simulink model "Subsystem"  (R2020a)
settings: Solver=FixedStepAuto  StartTime=0.0  StopTime=10.0  FixedStep=0.2  RelTol=1e-3
settings Model: Creator=Jake  LastModifiedBy=Jake
settings DataIOCC: SaveOutput=off  SaveTime=off

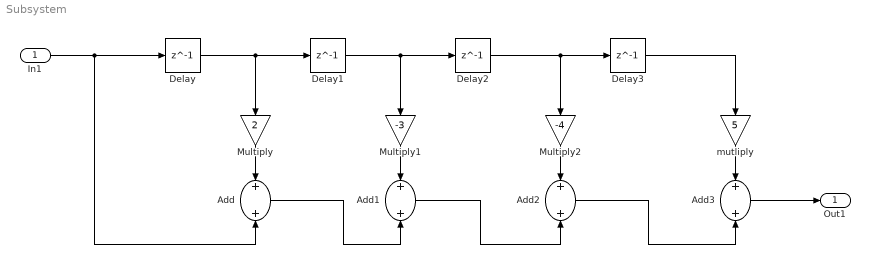
== system Subsystem ==
  In1 : Inport  OutDataTypeStr=double  PortDimensions=1  SampleTime=[0.20000000000000001,0]
  Add{,1..3} (4 alike) : Sum
  Delay{,1..3} (4 alike) : Delay  DelayLength=1
  Multiply : Gain  Gain=2
  Multiply1 : Gain  Gain=-3
  Multiply2 : Gain  Gain=-4
  mutliply : Gain  Gain=5
  Out1 : Outport  OutDataTypeStr=double  PortDimensions=1  SampleTime=[0.20000000000000001,0]
  wires:
  Multiply2/1 -> Add2/1
  Delay2/1 -> Multiply2/1, Delay3/1
  Delay/1 -> Delay1/1, Multiply/1
  Multiply1/1 -> Add1/1
  In1/1 -> Delay/1, Add/2
  Add/1 -> Add1/2
  Add2/1 -> Add3/2
  Delay1/1 -> Delay2/1, Multiply1/1
  mutliply/1 -> Add3/1
  Add1/1 -> Add2/2
  Multiply/1 -> Add/1
  Add3/1 -> Out1/1
  Delay3/1 -> mutliply/1
